simulink model "dinamica_inversa2015"  (R2015b)
settings: Solver=FixedStepAuto  SolverMode=SingleTasking  StartTime=0.0  StopTime=40  FixedStep=T  RelTol=1e-3
values from neighbouring files (symbols this model uses):
  Kd = 300*[1;1;1;1;1;1]    [PDpiuGravita.m]    (also in dinamica_inversa.m = diag([2*zita(1)*w_n(1) 2*zita(2)*w_n(2) 2*zita(3)*w_n(3) 2*z; mainPD.m = 500*ones(6,1))
  Kp = diag([500 500 500 50])    [Approccio1.m]    (also in Approccio2.m = 10*diag([50 50 50 5]); Approccio3.m = 10*diag([50 50 50 5]); InversioneCinematica.m = diag([100 100 10 10]); PDpiuGravita.m = 1200*[1;1;1;1;1;1])
  n = 6    [calcoloW.m]
undefined symbols (not defined in the file or in its folder): Bq, DirectDynamicsSim
settings Model: Creator=Giovanni  LastModifiedBy=Michele
settings DataIOCC: LimitDataPoints=off
settings DebuggingCC: AllowSymbolicDim=on  SFUnexpectedBacktrackingDiag=error  SFNoUnconditionalDefaultTransitionDiag=error
settings ModelReferenceCC: PropagateSignalLabelsOutOfModel=on
settings GRTTargetCC: TargetLangStandard=C99 (ISO)
settings ConfigComp: CovMetricSettings=dwe  CovHtmlReporting=off  CovSaveCumulativeToWorkspaceVar=off  CovSaveSingleToWorkspaceVar=off  CovModelRefEnable=Off  CovExternalEMLEnable=on

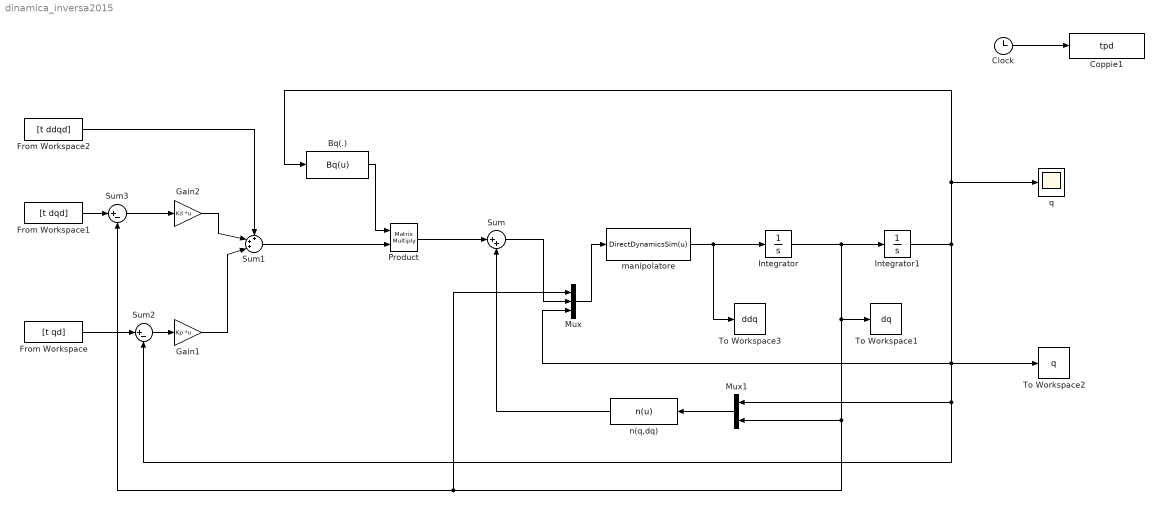
== system dinamica_inversa2015 ==
  Bq(.) : MATLABFcn  MATLABFcn=Bq(u)  OutputDimensions=[6 6]  Output1D=off
      mask Display: disp('Bq')
  Clock : Clock
  Coppie1 : ToWorkspace  VariableName=tpd  SampleTime=-1
  From Workspace : FromWorkspace  VariableName=[t qd]  SampleTime=0
  From Workspace1 : FromWorkspace  VariableName=[t dqd]  SampleTime=0
  From Workspace2 : FromWorkspace  VariableName=[t ddqd]  SampleTime=0
  Gain1 : Gain  Gain=Kp  Multiplication=Matrix(K*u)
  Gain2 : Gain  Gain=Kd  Multiplication=Matrix(K*u)
  Integrator : Integrator  InitialCondition=zeros(6,1)
  Integrator1 : Integrator  InitialCondition=zeros(6,1)
  Mux : Mux  Inputs=3
  Mux1 : Mux  Inputs=2
  Product : Product  Multiplication=Matrix(*)
  Sum : Sum  Inputs=|++
  Sum1 : Sum  Inputs=+++|
  Sum2 : Sum  Inputs=|+-
  Sum3 : Sum  Inputs=|+-
  To Workspace1 : ToWorkspace  VariableName=dq  SampleTime=-1
  To Workspace2 : ToWorkspace  VariableName=q  SampleTime=-1
  To Workspace3 : ToWorkspace  VariableName=ddq  SampleTime=-1
  manipolatore : MATLABFcn  MATLABFcn=DirectDynamicsSim(u)
      mask Display: disp ('DirectDynamicsSim')
  n(q,dq) : MATLABFcn  MATLABFcn=n(u)  Output1D=off
      mask Display: disp('n')
  q : Scope
  wires:
  Clock/1 -> Coppie1/1
  manipolatore/1 -> To Workspace3/1, Integrator/1
  Integrator1/1 -> Sum2/2, Mux1/1, Mux/3, To Workspace2/1, Bq(.)/1, q/1
  Integrator/1 -> Sum3/2, Mux/1, Mux1/2, To Workspace1/1, Integrator1/1
  Mux/1 -> manipolatore/1
  Sum/1 -> Mux/2
  n(q,dq)/1 -> Sum/2
  Gain1/1 -> Sum1/3
  Sum2/1 -> Gain1/1
  From Workspace/1 -> Sum2/1
  From Workspace1/1 -> Sum3/1
  Sum3/1 -> Gain2/1
  From Workspace2/1 -> Sum1/1
  Gain2/1 -> Sum1/2
  Bq(.)/1 -> Product/1
  Sum1/1 -> Product/2
  Product/1 -> Sum/1
  Mux1/1 -> n(q,dq)/1
